simulink model "node23_case_10kV_withLoad_v2"  (R2022b)
settings: Solver=VariableStepAuto  StartTime=0.0  StopTime=10  FixedStep=1e-6  RelTol=1e-5
InitFcn:
  | sw=5;
  | Lf=1.75e-3+3.5e-3;
  | %Lf=3.5e-3;
  | %Cf=2e-4;
  | f=10;
  | Cf=15e-6;
  | % L=1.75e-3/2;
  | % X=100*pi*L;
  | % R=2*X;
  | R=0.25;X=R/0.66;
  | L=X/100/pi;
  | Z=sqrt(R^2+X^2);
  | f = 30;
  | kp1=10;
  | ki1=100;
  | kp4=20;
  | ki4=100;
  | kp16=20;
  | ki16=100;
  | % 负载参数
  | R1L=0;
  | X1L=0;
  | R2L=652.4467;
  | X2L=276.0351;
  | R3L=804.5741;
  | X3L=256.7790;
  | R4L=760.9867;
  | X4L=234.6376;
  | R5L=818.7384;
  | X5L=266.9799;
  | R6L=671.1329;
  | X6L=170.1801;
  | R7L=883.7621;
  | X7L=178.8663;
  | R8L=388.3725;
  | X8L=158.3040;
  | R9L=817.4819;
  | X9L=268.6933;
  | R10L=849.4733;
  | X10L=254.8420;
  | R11L=407.8415;
  | X11L=165.8504;
  | R12L=NaN;  % Bus 12 无 R、X 数据，用 NaN 标记
  | X12L=NaN;
  | R13L=751.2339;
  | X13L=329.8428;
  | R14L=294.0393;
  | X14L=141.6929;
  | R15L=761.9027;
  | X15L=284.3908;
  | R16L=740.4040;
  | X16L=318.2438;
  | R17L=674.5784;
  | X17L=316.4689;
  | R18L=776.7449;
  | X18L=316.6080;
  | R19L=766.0423;
  | X19L=335.7994;
  | R20L=746.0545;
  | X20L=344.3329;
  | ... (+266 lines)
libraries: spsSeriesRLCBranchLib x210, slpidlib x45, spsControlledVoltageSourceLib x30, spsThreePhaseVIMeasurementLib x24, spsPower3phInstantaneousLib x13, spsAlphaBetaZerotoabcLib x9, spsCurrentMeasurementLib x6, spsGroundLib x2, spspowerguiLib x1
(part 3 of 8)

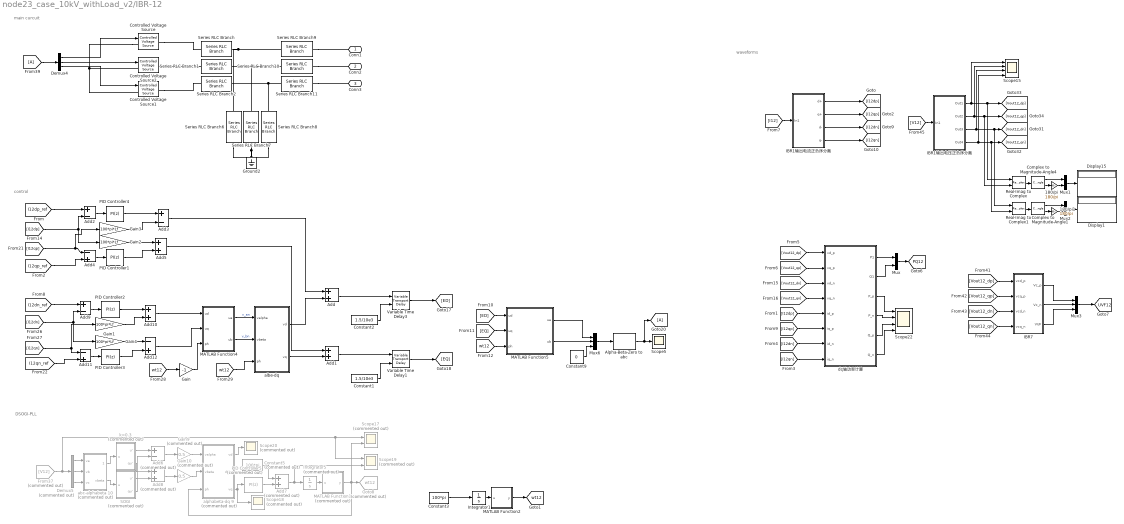
== system node23_case_10kV_withLoad_v2/IBR-12 ==
  note: waveforms
  note: DSOGI-PLL
  note: control
  note: main curcuit
  180/pi : Gain  Gain=180/pi
  180/pi1 : Gain  Gain=180/pi
  Add{,1,5,10} (4 alike) : Sum
  Add11 : Sum  Inputs=-+
  Add12 : Sum  Inputs=-+
  Add2 : Sum  Inputs=+-
  Add3 : Sum  Inputs=+-
  Add4 : Sum  Inputs=-+
  Add6 : Sum  Commented=on  Inputs=+-
  Add7 : Sum  Commented=on
  Add8 : Sum  Commented=on
  Add9 : Sum  Inputs=+-
  Alpha-Beta-Zero to abc : spsAlphaBetaZerotoabcLib/Alpha-Beta-Zero to abc
      settings: LibrarySourceBlock=|
      | sps_lib/Control/Alpha-Beta-Zero
      | to abc
  Complex to Magnitude-Angle1 : ComplexToMagnitudeAngle
  Complex to Magnitude-Angle4 : ComplexToMagnitudeAngle
  Constant1 : Constant  Value=1.5/10e3
  Constant2 : Constant  Value=1.5/10e3
  Constant3 : Constant  Value=100*pi
  Constant5 : Constant  Commented=on  Value=100*pi
  Constant9 : Constant  Value=0
  Controlled Voltage Source : spsControlledVoltageSourceLib/Controlled Voltage Source  Initialize=on  Source_Type=AC  Amplitude=0  Phase=0  Frequency=0  Measurements=None
  Controlled Voltage Source1 : spsControlledVoltageSourceLib/Controlled Voltage Source  Initialize=on  Source_Type=AC  Amplitude=0  Phase=0  Frequency=0  Measurements=None
  Controlled Voltage Source2 : spsControlledVoltageSourceLib/Controlled Voltage Source  Initialize=on  Source_Type=AC  Amplitude=0  Phase=0  Frequency=0  Measurements=None
  Demux4 : Demux  Outputs=3
  Demux5 : Demux  Commented=on  Outputs=3
  Display1 : Display
  Display15 : Display
  From37 : From  Commented=on  GotoTag=V12  TagVisibility=global
  From39 : From
  Gain : Gain  Gain=-1
  Gain{1..4} (4 alike) : Gain  Gain=100*pi*Lf
  Gain10 : Gain  Commented=on  Gain=0.5
  Gain9 : Gain  Commented=on  Gain=0.5
  Goto20 : Goto
  Goto8 : Goto  Commented=on  GotoTag=wt12  TagVisibility=global
  Ground2 : spsGroundLib/Ground  LConnTagsString=a
  IBR1输出电压正负序分离 : Subsystem
  IBR1输出电流正负序分离 : Subsystem
  IBR7 : MATLAB Function  TreatAsAtomicUnit=on
  Integrator1 : Integrator
  Integrator5 : Integrator  Commented=on
  MATLAB Function1 : MATLAB Function  Commented=on  TreatAsAtomicUnit=on
  MATLAB Function2 : MATLAB Function  TreatAsAtomicUnit=on
  MATLAB Function4 : MATLAB Function  TreatAsAtomicUnit=on
  MATLAB Function5 : MATLAB Function  TreatAsAtomicUnit=on
  Mux : Mux  Inputs=2
  Mux1 : Mux  Inputs=2
  Mux2 : Mux  Inputs=2
  Mux3 : Mux  Inputs=3
  Mux6 : Mux  Inputs=3
  PID Controller{1..4} (4 alike) : slpidlib/PID Controller  Controller=PI  Form=Parallel  TimeDomain=Discrete-time  UseExternalTs=off  SampleTime=-1  IntegratorMethod=Forward Euler  FilterMethod=Forward Euler  ControllerParametersSource=internal  P=kp1  I=ki1  UseKiTs=off  D=0  N=100  UseFilter=on  TunerSelectOption=Transfer Function Based (PID Tuner App)  InitialConditionSource=internal  InitialConditionForIntegrator=0  InitialConditionForFilter=0  DifferentiatorICPrevScaledInput=0  ExternalReset=none  TrackingMode=off  Kt=1  LimitOutput=off  SatLimitsSource=internal  UpperSaturationLimit=5  LowerSaturationLimit=-5  LinearizeAsGain=on  AntiWindupMode=none  Kb=1  LimitIntegrator=off  UpperIntegratorSaturationLimit=inf  LowerIntegratorSaturationLimit=-inf  POutMin=[]  POutMax=[]  IOutMin=[]  IOutMax=[]  DOutMin=[]  DOutMax=[]  NOutMin=[]  NOutMax=[]  SumOutMin=[]  SumOutMax=[]  SaturationOutMin=[]  SaturationOutMax=[]  PParamMin=[]  PParamMax=[]  IParamMin=[]  IParamMax=[]  DParamMin=[]  DParamMax=[]  NParamMin=[]  NParamMax=[]  KbParamMin=[]  KbParamMax=[]  KtParamMin=[]  KtParamMax=[]  KbOutMin=[]  KbOutMax=[]  KtOutMin=[]  KtOutMax=[]  IntegratorOutMin=[]  IntegratorOutMax=[]  FilterOutMin=[]  FilterOutMax=[]  SumI1OutMin=[]  SumI1OutMax=[]  SumI2OutMin=[]  SumI2OutMax=[]  SumI3OutMin=[]  SumI3OutMax=[]  SumI4OutMin=[]  SumI4OutMax=[]  SumDOutMin=[]  SumDOutMax=[]  DifferentiatorOutMin=[]  DifferentiatorOutMax=[]  FilterDiffOutCoefMin=[]  FilterDiffOutCoefMax=[]  ReciprocalOutMin=[]  ReciprocalOutMax=[]  SumDenOutMin=[]  SumDenOutMax=[]  SumNumOutMin=[]  SumNumOutMax=[]  DivideOutMin=[]  DivideOutMax=[]  UdiffTsProdOutMin=[]  UdiffTsProdOutMax=[]  NTsProdOutMin=[]  NTsProdOutMax=[]  UintegralTsProdOutMin=[]  UintegralTsProdOutMax=[]  UngainTsProdOutMin=[]  UngainTsProdOutMax=[]  ClampingZeroOutDataTypeStr=Inherit: Inherit via back propagation  ClampingZeroOutMin=[]  ClampingZeroOutMax=[]  FilterDenConstantOutDataTypeStr=Inherit: Inherit via back propagation  FilterDenConstantOutMin=[]  FilterDenConstantOutMax=[]  PCopyOutDataTypeStr=Inherit: Inherit via back propagation  PCopyOutMin=[]  PCopyOutMax=[]  NCopyOutDataTypeStr=Inherit: Inherit via back propagation  NCopyOutMin=[]  NCopyOutMax=[]  IntegratorContinuousStateAttributes=''  IntegratorStateMustResolveToSignalObject=off  IntegratorRTWStateStorageClass=Auto  FilterContinuousStateAttributes=''  FilterStateMustResolveToSignalObject=off  FilterRTWStateStorageClass=Auto  ParallelPVariant=InternalParameters  IdealPVariant=Disabled  IVariant=InternalParameters  DVariant=Disabled  IntegratorVariant=Discrete  SatVariant=Disabled  AWVariant=Passthrough  PCopyVariant=Disabled  TRVariant=Disabled  FdbkBlocksVariant=Forward  IdealPFdbkVariant=Disabled  SatFdbkVariant=Disabled  DerivativeFilterVariant=Disabled  NVariant=Disabled  NCopyVariant=Disabled_SignalSpec  FilterICVariant=Disabled  IntegratorICVariant=InternalICs  ExternalResetVariant=Disabled  TRSumVariant=Passthrough  SumFdbkVariant=Disabled  SumVariant=Sum_PI  TsampFilterVariant=InternalTs  TsampNgainVariant=Passthrough  TsampIntegralVariant=Passthrough  ExternalSaturationOutDataTypeStr=Inherit: Same as second input
  PID Controller5 : slpidlib/PID Controller  Commented=on  Controller=PI  Form=Parallel  TimeDomain=Discrete-time  UseExternalTs=off  SampleTime=-1  IntegratorMethod=Forward Euler  FilterMethod=Forward Euler  ControllerParametersSource=internal  P=1  I=3  UseKiTs=off  D=0  N=100  UseFilter=on  TunerSelectOption=Transfer Function Based (PID Tuner App)  InitialConditionSource=internal  InitialConditionForIntegrator=0  InitialConditionForFilter=0  DifferentiatorICPrevScaledInput=0  ExternalReset=none  TrackingMode=off  Kt=1  LimitOutput=off  SatLimitsSource=internal  UpperSaturationLimit=inf  LowerSaturationLimit=-inf  LinearizeAsGain=on  AntiWindupMode=none  Kb=1  LimitIntegrator=off  UpperIntegratorSaturationLimit=inf  LowerIntegratorSaturationLimit=-inf  POutMin=[]  POutMax=[]  IOutMin=[]  IOutMax=[]  DOutMin=[]  DOutMax=[]  NOutMin=[]  NOutMax=[]  SumOutMin=[]  SumOutMax=[]  SaturationOutMin=[]  SaturationOutMax=[]  PParamMin=[]  PParamMax=[]  IParamMin=[]  IParamMax=[]  DParamMin=[]  DParamMax=[]  NParamMin=[]  NParamMax=[]  KbParamMin=[]  KbParamMax=[]  KtParamMin=[]  KtParamMax=[]  KbOutMin=[]  KbOutMax=[]  KtOutMin=[]  KtOutMax=[]  IntegratorOutMin=[]  IntegratorOutMax=[]  FilterOutMin=[]  FilterOutMax=[]  SumI1OutMin=[]  SumI1OutMax=[]  SumI2OutMin=[]  SumI2OutMax=[]  SumI3OutMin=[]  SumI3OutMax=[]  SumI4OutMin=[]  SumI4OutMax=[]  SumDOutMin=[]  SumDOutMax=[]  DifferentiatorOutMin=[]  DifferentiatorOutMax=[]  FilterDiffOutCoefMin=[]  FilterDiffOutCoefMax=[]  ReciprocalOutMin=[]  ReciprocalOutMax=[]  SumDenOutMin=[]  SumDenOutMax=[]  SumNumOutMin=[]  SumNumOutMax=[]  DivideOutMin=[]  DivideOutMax=[]  UdiffTsProdOutMin=[]  UdiffTsProdOutMax=[]  NTsProdOutMin=[]  NTsProdOutMax=[]  UintegralTsProdOutMin=[]  UintegralTsProdOutMax=[]  UngainTsProdOutMin=[]  UngainTsProdOutMax=[]  ClampingZeroOutDataTypeStr=Inherit: Inherit via back propagation  ClampingZeroOutMin=[]  ClampingZeroOutMax=[]  FilterDenConstantOutDataTypeStr=Inherit: Inherit via back propagation  FilterDenConstantOutMin=[]  FilterDenConstantOutMax=[]  PCopyOutDataTypeStr=Inherit: Inherit via back propagation  PCopyOutMin=[]  PCopyOutMax=[]  NCopyOutDataTypeStr=Inherit: Inherit via back propagation  NCopyOutMin=[]  NCopyOutMax=[]  IntegratorContinuousStateAttributes=''  IntegratorStateMustResolveToSignalObject=off  IntegratorRTWStateStorageClass=Auto  FilterContinuousStateAttributes=''  FilterStateMustResolveToSignalObject=off  FilterRTWStateStorageClass=Auto  ParallelPVariant=InternalParameters  IdealPVariant=Disabled  IVariant=InternalParameters  DVariant=Disabled  IntegratorVariant=Discrete  SatVariant=Disabled  AWVariant=Passthrough  PCopyVariant=Disabled  TRVariant=Disabled  FdbkBlocksVariant=Forward  IdealPFdbkVariant=Disabled  SatFdbkVariant=Disabled  DerivativeFilterVariant=Disabled  NVariant=Disabled  NCopyVariant=Disabled_SignalSpec  FilterICVariant=Disabled  IntegratorICVariant=InternalICs  ExternalResetVariant=Disabled  TRSumVariant=Passthrough  SumFdbkVariant=Disabled  SumVariant=Sum_PI  TsampFilterVariant=InternalTs  TsampNgainVariant=Passthrough  TsampIntegralVariant=Passthrough  ExternalSaturationOutDataTypeStr=Inherit: Same as second input
  Real-Imag to Complex : RealImagToComplex
  Real-Imag to Complex1 : RealImagToComplex
  SOGI : Subsystem  Commented=on
  Scope15 : Scope  NumInputPorts=4
  Scope17 : Scope  Commented=on  NumInputPorts=2
  Scope18 : Scope  Commented=on
  Scope19 : Scope  Commented=on  NumInputPorts=2
  Scope20 : Scope  Commented=on
  Scope22 : Scope  NumInputPorts=4
  Scope5 : Scope
  Series RLC Branch : spsSeriesRLCBranchLib/Series RLC Branch  LConnTagsString=__new0  RConnTagsString=__new0  BranchType=L  Resistance=1  Inductance=3.5e-3  SetiL0=off  InitialCurrent=0  Capacitance=1e-6  Setx0=off  InitialVoltage=0  Measurements=None
  Series RLC Branch1 : spsSeriesRLCBranchLib/Series RLC Branch  LConnTagsString=__new0  RConnTagsString=__new0  BranchType=L  Resistance=1  Inductance=3.5e-3  SetiL0=off  InitialCurrent=0  Capacitance=1e-6  Setx0=off  InitialVoltage=0  Measurements=None
  Series RLC Branch10 : spsSeriesRLCBranchLib/Series RLC Branch  LConnTagsString=__new0  RConnTagsString=__new0  BranchType=L  Resistance=1  Inductance=1.75e-3  SetiL0=off  InitialCurrent=0  Capacitance=1e-6  Setx0=off  InitialVoltage=0  Measurements=None
  Series RLC Branch11 : spsSeriesRLCBranchLib/Series RLC Branch  LConnTagsString=__new0  RConnTagsString=__new0  BranchType=L  Resistance=1  Inductance=1.75e-3  SetiL0=off  InitialCurrent=0  Capacitance=1e-6  Setx0=off  InitialVoltage=0  Measurements=None
  Series RLC Branch2 : spsSeriesRLCBranchLib/Series RLC Branch  LConnTagsString=__new0  RConnTagsString=__new0  BranchType=L  Resistance=1  Inductance=3.5e-3  SetiL0=off  InitialCurrent=0  Capacitance=1e-6  Setx0=off  InitialVoltage=0  Measurements=None
  Series RLC Branch6 : spsSeriesRLCBranchLib/Series RLC Branch  LConnTagsString=__new0  RConnTagsString=__new0  BranchType=RC  Resistance=5  Inductance=500e-6  SetiL0=off  InitialCurrent=0  Capacitance=Cf  Setx0=off  InitialVoltage=0  Measurements=None
  Series RLC Branch7 : spsSeriesRLCBranchLib/Series RLC Branch  LConnTagsString=__new0  RConnTagsString=__new0  BranchType=RC  Resistance=5  Inductance=500e-6  SetiL0=off  InitialCurrent=0  Capacitance=Cf  Setx0=off  InitialVoltage=0  Measurements=None
  Series RLC Branch8 : spsSeriesRLCBranchLib/Series RLC Branch  LConnTagsString=__new0  RConnTagsString=__new0  BranchType=RC  Resistance=5  Inductance=500e-6  SetiL0=off  InitialCurrent=0  Capacitance=Cf  Setx0=off  InitialVoltage=0  Measurements=None
  Series RLC Branch9 : spsSeriesRLCBranchLib/Series RLC Branch  LConnTagsString=__new0  RConnTagsString=__new0  BranchType=L  Resistance=1  Inductance=1.75e-3  SetiL0=off  InitialCurrent=0  Capacitance=1e-6  Setx0=off  InitialVoltage=0  Measurements=None
  Variable Time Delay1 : VariableTransportDelay  MaximumDelay=10  PadeOrder=2
  Variable Time Delay3 : VariableTransportDelay  MaximumDelay=10  PadeOrder=2
  abc-alphabeta 10 : MATLAB Function  Commented=on  TreatAsAtomicUnit=on
  albe-dq : MATLAB Function  TreatAsAtomicUnit=on
  alphabeta-dq 9 : MATLAB Function  Commented=on  TreatAsAtomicUnit=on
  dq轴功率计算 : MATLAB Function  TreatAsAtomicUnit=on
  k=0.3 : Subsystem  Commented=on
  Conn1 : PMIOPort  Side=Right
  Conn2 : PMIOPort  Port=2  Side=Right
  Conn3 : PMIOPort  Port=3  Side=Right
  tag scope: PQ12=global, UVF12=global, wt12=global
  wires:
  IBR1输出电压正负序分离/4(Out4) -> [Vout12_qn], Real-Imag to Complex1/2, Scope15/4
  Complex to Magnitude-Angle1/1 -> Mux2/1
  Complex to Magnitude-Angle1/2 -> 180/pi1/1
  Real-Imag to Complex1/1 -> Complex to Magnitude-Angle1/1
  180/pi1/1 -> Mux2/2
  Mux2/1 -> Display1/1
  IBR1输出电压正负序分离/1(Out1) -> Scope15/1, [Vout12_dp], Real-Imag to Complex/1
  Mux1/1 -> Display15/1
  180/pi/1 -> Mux1/2
  Real-Imag to Complex/1 -> Complex to Magnitude-Angle4/1
  Complex to Magnitude-Angle4/2 -> 180/pi/1
  Complex to Magnitude-Angle4/1 -> Mux1/1
  Mux/1 -> [PQ12]
  [I12dn] -> dq轴功率计算/7(id_n)
  [I12qp] -> dq轴功率计算/6(iq_p)
  [I12dp] -> dq轴功率计算/5(id_p)
  [Vout12_qn] -> dq轴功率计算/4(vq_n)
  [Vout12_dn] -> dq轴功率计算/3(vd_n)
  [Vout12_qp] -> dq轴功率计算/2(vq_p)
  [I12qn] -> dq轴功率计算/8(iq_n)
  [Vout12_dp] -> dq轴功率计算/1(vd_p)
  dq轴功率计算/2(Q1) -> Mux/2
  dq轴功率计算/3(P_p) -> Scope22/1
  dq轴功率计算/5(Q_p) -> Scope22/3
  dq轴功率计算/4(P_n) -> Scope22/2
  dq轴功率计算/6(Q_n) -> Scope22/4
  dq轴功率计算/1(P1) -> Mux/1
  [wt12] -> Gain/1
  MATLAB Function4/1(ua) -> albe-dq/1(valpha)  "v_an"
  [I12qn] -> Add11/1, Gain1/1
  [I12dn] -> Gain4/1, Add9/2
  PID Controller1/1 -> Add5/2
  albe-dq/2(vq) -> Add1/2
  Gain1/1 -> Add10/2
  Add5/1 -> Add1/1
  albe-dq/1(vd) -> Add/2
  Gain2/1 -> Add5/1
  [I12qp] -> Add4/1, Gain3/1
  [wt12] -> albe-dq/3(ph)
  PID Controller4/1 -> Add3/1
  Gain3/1 -> Add3/2
  Add4/1 -> PID Controller1/1
  [ED] -> MATLAB Function5/1(ud)
  Add11/1 -> PID Controller3/1
  Add10/1 -> MATLAB Function4/1(ud)
  MATLAB Function4/2(ub) -> albe-dq/2(vbeta)  "v_bn"
  MATLAB Function5/2(ub) -> Mux6/2
  Add9/1 -> PID Controller2/1
  Gain/1 -> MATLAB Function4/3(ph)
  Gain4/1 -> Add12/1
  [I12dp] -> Add2/2, Gain2/1
  PID Controller2/1 -> Add10/1
  PID Controller3/1 -> Add12/2
  Add3/1 -> Add/1
  [wt12] -> MATLAB Function5/3(ph)
  Add12/1 -> MATLAB Function4/2(uq)
  [EQ] -> MATLAB Function5/2(uq)
  [Vout12_qn] -> IBR7/4(vcq_n)
  [Vout12_dp] -> IBR7/1(vcd_p)
  [Vout12_qp] -> IBR7/2(vcq_p)
  [Vout12_dn] -> IBR7/3(vcd_n)
  [I12] -> IBR1输出电流正负序分离/1(In1)
  IBR1输出电流正负序分离/1(d+) -> [I12dp]
  IBR1输出电压正负序分离/2(Out2) -> [Vout12_qp], Real-Imag to Complex/2, Scope15/2
  [V12] -> IBR1输出电压正负序分离/1(In1)
  IBR1输出电流正负序分离/4(q-) -> [I12qn]
  IBR1输出电压正负序分离/3(Out3) -> Scope15/3, [Vout12_dn], Real-Imag to Complex1/1
  IBR7/2(Vc_n) -> Mux3/2
  IBR7/1(Vc_p) -> Mux3/1
  IBR7/3(VUF) -> Mux3/3
  Mux3/1 -> [UVF12]
  Add2/1 -> PID Controller4/1
  MATLAB Function5/1(ua) -> Mux6/1
  Mux6/1 -> Alpha-Beta-Zero to abc/1
  Alpha-Beta-Zero to abc/1 -> Goto20/1, Scope5/1
  Constant9/1 -> Mux6/3
  From39/1 -> Demux4/1
  Demux4/2 -> Controlled Voltage Source2/1
  Demux4/3 -> Controlled Voltage Source1/1
  Demux4/1 -> Controlled Voltage Source/1
  [I12qn_ref] -> Add11/2
  [I12dn_ref] -> Add9/1
  [I12qp_ref] -> Add4/2
  [I12dp_ref] -> Add2/1
  IBR1输出电流正负序分离/2(q+) -> [I12qp]
  IBR1输出电流正负序分离/3(d-) -> [I12dn]
  Add/1 -> Variable Time Delay3/1
  Constant2/1 -> Variable Time Delay3/2
  Variable Time Delay3/1 -> [ED]
  Constant1/1 -> Variable Time Delay1/2
  Add1/1 -> Variable Time Delay1/1
  Variable Time Delay1/1 -> [EQ]
  Add8/1 -> Gain10/1
  Gain9/1 -> alphabeta-dq 9/1(valpha)
  Integrator5/1 -> MATLAB Function1/1(u)
  MATLAB Function1/1(y) -> Goto8/1, Scope17/2, alphabeta-dq 9/3(ph)
  Constant5/1 -> Add7/1
  alphabeta-dq 9/1(vd) -> Scope20/1
  From37/1 -> Scope19/1, Scope17/1, Demux5/1
  Gain10/1 -> alphabeta-dq 9/2(vbeta)
  alphabeta-dq 9/3(vq) -> PID Controller5/1, Scope18/1
  SOGI/1(u') -> Add8/2
  Add7/1 -> Integrator5/1, Scope19/2
  k=0.3/1(u') -> Add6/1
  Add6/1 -> Gain9/1
  abc-alphabeta 10/1(valpha) -> k=0.3/1(u)
  Demux5/2 -> abc-alphabeta 10/2(vb)
  Demux5/1 -> abc-alphabeta 10/1(va)
  k=0.3/2(qu') -> Add8/1
  Demux5/3 -> abc-alphabeta 10/3(vc)
  SOGI/2(qu') -> Add6/2
  abc-alphabeta 10/2(vbeta) -> SOGI/1(u)
  PID Controller5/1 -> Add7/2
  Constant3/1 -> Integrator1/1
  MATLAB Function2/1(y) -> [wt12]
  Integrator1/1 -> MATLAB Function2/1(u)
  connections:
  Series RLC Branch9/RConn1 -- Conn1/RConn1
  Series RLC Branch10/RConn1 -- Conn2/RConn1
  Series RLC Branch11/RConn1 -- Conn3/RConn1
  Controlled Voltage Source/RConn1 -- Series RLC Branch/LConn1
  Series RLC Branch8/RConn1 -- Series RLC Branch6/RConn1 -- Series RLC Branch7/RConn1 -- Ground2/LConn1
  Controlled Voltage Source1/RConn1 -- Series RLC Branch2/LConn1
  Controlled Voltage Source2/RConn1 -- Series RLC Branch1/LConn1
  Series RLC Branch9/LConn1 -- Series RLC Branch6/LConn1 -- Series RLC Branch/RConn1
  Series RLC Branch10/LConn1 -- Series RLC Branch1/RConn1 -- Series RLC Branch7/LConn1
  Series RLC Branch11/LConn1 -- Series RLC Branch2/RConn1 -- Series RLC Branch8/LConn1
  Controlled Voltage Source/LConn1 -- Controlled Voltage Source2/LConn1 -- Controlled Voltage Source1/LConn1

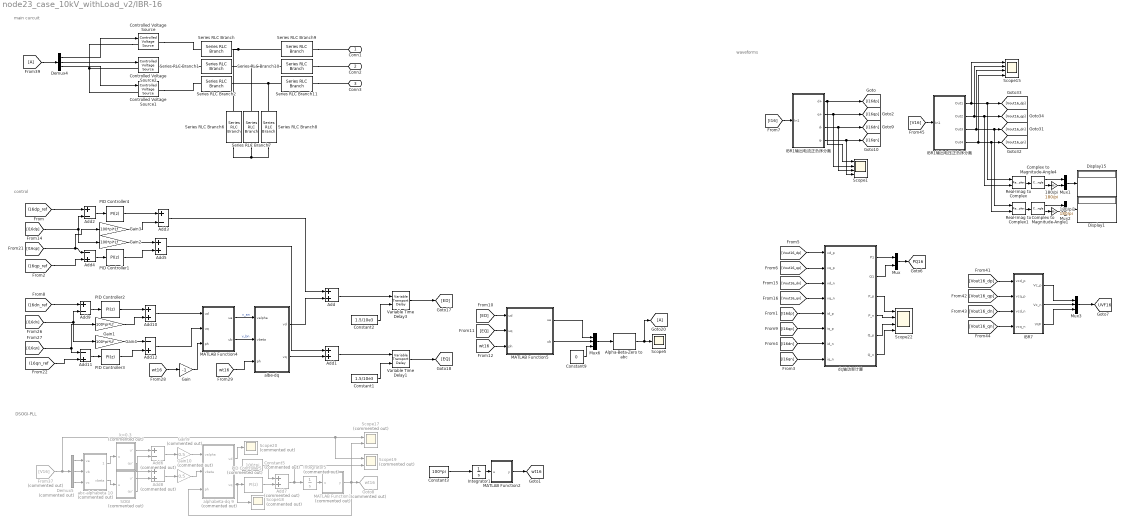
== system node23_case_10kV_withLoad_v2/IBR-16 ==
  note: waveforms
  note: DSOGI-PLL
  note: control
  note: main curcuit
  180/pi : Gain  Gain=180/pi
  180/pi1 : Gain  Gain=180/pi
  Add{,1,5,10} (4 alike) : Sum
  Add11 : Sum  Inputs=-+
  Add12 : Sum  Inputs=-+
  Add2 : Sum  Inputs=+-
  Add3 : Sum  Inputs=+-
  Add4 : Sum  Inputs=-+
  Add6 : Sum  Commented=on  Inputs=+-
  Add7 : Sum  Commented=on
  Add8 : Sum  Commented=on
  Add9 : Sum  Inputs=+-
  Alpha-Beta-Zero to abc : spsAlphaBetaZerotoabcLib/Alpha-Beta-Zero to abc
      settings: LibrarySourceBlock=|
      | sps_lib/Control/Alpha-Beta-Zero
      | to abc
  Complex to Magnitude-Angle1 : ComplexToMagnitudeAngle
  Complex to Magnitude-Angle4 : ComplexToMagnitudeAngle
  Constant1 : Constant  Value=1.5/10e3
  Constant2 : Constant  Value=1.5/10e3
  Constant3 : Constant  Value=100*pi
  Constant5 : Constant  Commented=on  Value=100*pi
  Constant9 : Constant  Value=0
  Controlled Voltage Source : spsControlledVoltageSourceLib/Controlled Voltage Source  Initialize=on  Source_Type=AC  Amplitude=0  Phase=0  Frequency=0  Measurements=None
  Controlled Voltage Source1 : spsControlledVoltageSourceLib/Controlled Voltage Source  Initialize=on  Source_Type=AC  Amplitude=0  Phase=0  Frequency=0  Measurements=None
  Controlled Voltage Source2 : spsControlledVoltageSourceLib/Controlled Voltage Source  Initialize=on  Source_Type=AC  Amplitude=0  Phase=0  Frequency=0  Measurements=None
  Demux4 : Demux  Outputs=3
  Demux5 : Demux  Commented=on  Outputs=3
  Display1 : Display
  Display15 : Display
  From37 : From  Commented=on  GotoTag=V16  TagVisibility=global
  From39 : From
  Gain : Gain  Gain=-1
  Gain{1..4} (4 alike) : Gain  Gain=100*pi*Lf
  Gain10 : Gain  Commented=on  Gain=0.5
  Gain9 : Gain  Commented=on  Gain=0.5
  Goto20 : Goto
  Goto8 : Goto  Commented=on  GotoTag=wt16  TagVisibility=global
  IBR1输出电压正负序分离 : Subsystem
  IBR1输出电流正负序分离 : Subsystem
  IBR7 : MATLAB Function  TreatAsAtomicUnit=on
  Integrator1 : Integrator
  Integrator5 : Integrator  Commented=on
  MATLAB Function1 : MATLAB Function  Commented=on  TreatAsAtomicUnit=on
  MATLAB Function2 : MATLAB Function  TreatAsAtomicUnit=on
  MATLAB Function4 : MATLAB Function  TreatAsAtomicUnit=on
  MATLAB Function5 : MATLAB Function  TreatAsAtomicUnit=on
  Mux : Mux  Inputs=2
  Mux1 : Mux  Inputs=2
  Mux2 : Mux  Inputs=2
  Mux3 : Mux  Inputs=3
  Mux6 : Mux  Inputs=3
  PID Controller{1..4} (4 alike) : slpidlib/PID Controller  Controller=PI  Form=Parallel  TimeDomain=Discrete-time  UseExternalTs=off  SampleTime=-1  IntegratorMethod=Forward Euler  FilterMethod=Forward Euler  ControllerParametersSource=internal  P=kp16  I=ki16  UseKiTs=off  D=0  N=100  UseFilter=on  TunerSelectOption=Transfer Function Based (PID Tuner App)  InitialConditionSource=internal  InitialConditionForIntegrator=0  InitialConditionForFilter=0  DifferentiatorICPrevScaledInput=0  ExternalReset=none  TrackingMode=off  Kt=1  LimitOutput=off  SatLimitsSource=internal  UpperSaturationLimit=5  LowerSaturationLimit=-5  LinearizeAsGain=on  AntiWindupMode=none  Kb=1  LimitIntegrator=off  UpperIntegratorSaturationLimit=inf  LowerIntegratorSaturationLimit=-inf  POutMin=[]  POutMax=[]  IOutMin=[]  IOutMax=[]  DOutMin=[]  DOutMax=[]  NOutMin=[]  NOutMax=[]  SumOutMin=[]  SumOutMax=[]  SaturationOutMin=[]  SaturationOutMax=[]  PParamMin=[]  PParamMax=[]  IParamMin=[]  IParamMax=[]  DParamMin=[]  DParamMax=[]  NParamMin=[]  NParamMax=[]  KbParamMin=[]  KbParamMax=[]  KtParamMin=[]  KtParamMax=[]  KbOutMin=[]  KbOutMax=[]  KtOutMin=[]  KtOutMax=[]  IntegratorOutMin=[]  IntegratorOutMax=[]  FilterOutMin=[]  FilterOutMax=[]  SumI1OutMin=[]  SumI1OutMax=[]  SumI2OutMin=[]  SumI2OutMax=[]  SumI3OutMin=[]  SumI3OutMax=[]  SumI4OutMin=[]  SumI4OutMax=[]  SumDOutMin=[]  SumDOutMax=[]  DifferentiatorOutMin=[]  DifferentiatorOutMax=[]  FilterDiffOutCoefMin=[]  FilterDiffOutCoefMax=[]  ReciprocalOutMin=[]  ReciprocalOutMax=[]  SumDenOutMin=[]  SumDenOutMax=[]  SumNumOutMin=[]  SumNumOutMax=[]  DivideOutMin=[]  DivideOutMax=[]  UdiffTsProdOutMin=[]  UdiffTsProdOutMax=[]  NTsProdOutMin=[]  NTsProdOutMax=[]  UintegralTsProdOutMin=[]  UintegralTsProdOutMax=[]  UngainTsProdOutMin=[]  UngainTsProdOutMax=[]  ClampingZeroOutDataTypeStr=Inherit: Inherit via back propagation  ClampingZeroOutMin=[]  ClampingZeroOutMax=[]  FilterDenConstantOutDataTypeStr=Inherit: Inherit via back propagation  FilterDenConstantOutMin=[]  FilterDenConstantOutMax=[]  PCopyOutDataTypeStr=Inherit: Inherit via back propagation  PCopyOutMin=[]  PCopyOutMax=[]  NCopyOutDataTypeStr=Inherit: Inherit via back propagation  NCopyOutMin=[]  NCopyOutMax=[]  IntegratorContinuousStateAttributes=''  IntegratorStateMustResolveToSignalObject=off  IntegratorRTWStateStorageClass=Auto  FilterContinuousStateAttributes=''  FilterStateMustResolveToSignalObject=off  FilterRTWStateStorageClass=Auto  ParallelPVariant=InternalParameters  IdealPVariant=Disabled  IVariant=InternalParameters  DVariant=Disabled  IntegratorVariant=Discrete  SatVariant=Disabled  AWVariant=Passthrough  PCopyVariant=Disabled  TRVariant=Disabled  FdbkBlocksVariant=Forward  IdealPFdbkVariant=Disabled  SatFdbkVariant=Disabled  DerivativeFilterVariant=Disabled  NVariant=Disabled  NCopyVariant=Disabled_SignalSpec  FilterICVariant=Disabled  IntegratorICVariant=InternalICs  ExternalResetVariant=Disabled  TRSumVariant=Passthrough  SumFdbkVariant=Disabled  SumVariant=Sum_PI  TsampFilterVariant=InternalTs  TsampNgainVariant=Passthrough  TsampIntegralVariant=Passthrough  ExternalSaturationOutDataTypeStr=Inherit: Same as second input
  PID Controller5 : slpidlib/PID Controller  Commented=on  Controller=PI  Form=Parallel  TimeDomain=Discrete-time  UseExternalTs=off  SampleTime=-1  IntegratorMethod=Forward Euler  FilterMethod=Forward Euler  ControllerParametersSource=internal  P=1  I=3  UseKiTs=off  D=0  N=100  UseFilter=on  TunerSelectOption=Transfer Function Based (PID Tuner App)  InitialConditionSource=internal  InitialConditionForIntegrator=0  InitialConditionForFilter=0  DifferentiatorICPrevScaledInput=0  ExternalReset=none  TrackingMode=off  Kt=1  LimitOutput=off  SatLimitsSource=internal  UpperSaturationLimit=inf  LowerSaturationLimit=-inf  LinearizeAsGain=on  AntiWindupMode=none  Kb=1  LimitIntegrator=off  UpperIntegratorSaturationLimit=inf  LowerIntegratorSaturationLimit=-inf  POutMin=[]  POutMax=[]  IOutMin=[]  IOutMax=[]  DOutMin=[]  DOutMax=[]  NOutMin=[]  NOutMax=[]  SumOutMin=[]  SumOutMax=[]  SaturationOutMin=[]  SaturationOutMax=[]  PParamMin=[]  PParamMax=[]  IParamMin=[]  IParamMax=[]  DParamMin=[]  DParamMax=[]  NParamMin=[]  NParamMax=[]  KbParamMin=[]  KbParamMax=[]  KtParamMin=[]  KtParamMax=[]  KbOutMin=[]  KbOutMax=[]  KtOutMin=[]  KtOutMax=[]  IntegratorOutMin=[]  IntegratorOutMax=[]  FilterOutMin=[]  FilterOutMax=[]  SumI1OutMin=[]  SumI1OutMax=[]  SumI2OutMin=[]  SumI2OutMax=[]  SumI3OutMin=[]  SumI3OutMax=[]  SumI4OutMin=[]  SumI4OutMax=[]  SumDOutMin=[]  SumDOutMax=[]  DifferentiatorOutMin=[]  DifferentiatorOutMax=[]  FilterDiffOutCoefMin=[]  FilterDiffOutCoefMax=[]  ReciprocalOutMin=[]  ReciprocalOutMax=[]  SumDenOutMin=[]  SumDenOutMax=[]  SumNumOutMin=[]  SumNumOutMax=[]  DivideOutMin=[]  DivideOutMax=[]  UdiffTsProdOutMin=[]  UdiffTsProdOutMax=[]  NTsProdOutMin=[]  NTsProdOutMax=[]  UintegralTsProdOutMin=[]  UintegralTsProdOutMax=[]  UngainTsProdOutMin=[]  UngainTsProdOutMax=[]  ClampingZeroOutDataTypeStr=Inherit: Inherit via back propagation  ClampingZeroOutMin=[]  ClampingZeroOutMax=[]  FilterDenConstantOutDataTypeStr=Inherit: Inherit via back propagation  FilterDenConstantOutMin=[]  FilterDenConstantOutMax=[]  PCopyOutDataTypeStr=Inherit: Inherit via back propagation  PCopyOutMin=[]  PCopyOutMax=[]  NCopyOutDataTypeStr=Inherit: Inherit via back propagation  NCopyOutMin=[]  NCopyOutMax=[]  IntegratorContinuousStateAttributes=''  IntegratorStateMustResolveToSignalObject=off  IntegratorRTWStateStorageClass=Auto  FilterContinuousStateAttributes=''  FilterStateMustResolveToSignalObject=off  FilterRTWStateStorageClass=Auto  ParallelPVariant=InternalParameters  IdealPVariant=Disabled  IVariant=InternalParameters  DVariant=Disabled  IntegratorVariant=Discrete  SatVariant=Disabled  AWVariant=Passthrough  PCopyVariant=Disabled  TRVariant=Disabled  FdbkBlocksVariant=Forward  IdealPFdbkVariant=Disabled  SatFdbkVariant=Disabled  DerivativeFilterVariant=Disabled  NVariant=Disabled  NCopyVariant=Disabled_SignalSpec  FilterICVariant=Disabled  IntegratorICVariant=InternalICs  ExternalResetVariant=Disabled  TRSumVariant=Passthrough  SumFdbkVariant=Disabled  SumVariant=Sum_PI  TsampFilterVariant=InternalTs  TsampNgainVariant=Passthrough  TsampIntegralVariant=Passthrough  ExternalSaturationOutDataTypeStr=Inherit: Same as second input
  Real-Imag to Complex : RealImagToComplex
  Real-Imag to Complex1 : RealImagToComplex
  SOGI : Subsystem  Commented=on
  Scope1 : Scope  NumInputPorts=4
  Scope15 : Scope  NumInputPorts=4
  Scope17 : Scope  Commented=on  NumInputPorts=2
  Scope18 : Scope  Commented=on
  Scope19 : Scope  Commented=on  NumInputPorts=2
  Scope20 : Scope  Commented=on
  Scope22 : Scope  NumInputPorts=4
  Scope5 : Scope
  Series RLC Branch : spsSeriesRLCBranchLib/Series RLC Branch  LConnTagsString=__new0  RConnTagsString=__new0  BranchType=L  Resistance=1  Inductance=3.5e-3  SetiL0=off  InitialCurrent=0  Capacitance=1e-6  Setx0=off  InitialVoltage=0  Measurements=None
  Series RLC Branch1 : spsSeriesRLCBranchLib/Series RLC Branch  LConnTagsString=__new0  RConnTagsString=__new0  BranchType=L  Resistance=1  Inductance=3.5e-3  SetiL0=off  InitialCurrent=0  Capacitance=1e-6  Setx0=off  InitialVoltage=0  Measurements=None
  Series RLC Branch10 : spsSeriesRLCBranchLib/Series RLC Branch  LConnTagsString=__new0  RConnTagsString=__new0  BranchType=L  Resistance=1  Inductance=1.75e-3  SetiL0=off  InitialCurrent=0  Capacitance=1e-6  Setx0=off  InitialVoltage=0  Measurements=None
  Series RLC Branch11 : spsSeriesRLCBranchLib/Series RLC Branch  LConnTagsString=__new0  RConnTagsString=__new0  BranchType=L  Resistance=1  Inductance=1.75e-3  SetiL0=off  InitialCurrent=0  Capacitance=1e-6  Setx0=off  InitialVoltage=0  Measurements=None
  Series RLC Branch2 : spsSeriesRLCBranchLib/Series RLC Branch  LConnTagsString=__new0  RConnTagsString=__new0  BranchType=L  Resistance=1  Inductance=3.5e-3  SetiL0=off  InitialCurrent=0  Capacitance=1e-6  Setx0=off  InitialVoltage=0  Measurements=None
  Series RLC Branch6 : spsSeriesRLCBranchLib/Series RLC Branch  LConnTagsString=__new0  RConnTagsString=__new0  BranchType=RC  Resistance=5  Inductance=500e-6  SetiL0=off  InitialCurrent=0  Capacitance=Cf  Setx0=off  InitialVoltage=0  Measurements=None
  Series RLC Branch7 : spsSeriesRLCBranchLib/Series RLC Branch  LConnTagsString=__new0  RConnTagsString=__new0  BranchType=RC  Resistance=5  Inductance=500e-6  SetiL0=off  InitialCurrent=0  Capacitance=Cf  Setx0=off  InitialVoltage=0  Measurements=None
  Series RLC Branch8 : spsSeriesRLCBranchLib/Series RLC Branch  LConnTagsString=__new0  RConnTagsString=__new0  BranchType=RC  Resistance=5  Inductance=500e-6  SetiL0=off  InitialCurrent=0  Capacitance=Cf  Setx0=off  InitialVoltage=0  Measurements=None
  Series RLC Branch9 : spsSeriesRLCBranchLib/Series RLC Branch  LConnTagsString=__new0  RConnTagsString=__new0  BranchType=L  Resistance=1  Inductance=1.75e-3  SetiL0=off  InitialCurrent=0  Capacitance=1e-6  Setx0=off  InitialVoltage=0  Measurements=None
  Variable Time Delay1 : VariableTransportDelay  MaximumDelay=10  PadeOrder=2
  Variable Time Delay3 : VariableTransportDelay  MaximumDelay=10  PadeOrder=2
  abc-alphabeta 10 : MATLAB Function  Commented=on  TreatAsAtomicUnit=on
  albe-dq : MATLAB Function  TreatAsAtomicUnit=on
  alphabeta-dq 9 : MATLAB Function  Commented=on  TreatAsAtomicUnit=on
  dq轴功率计算 : MATLAB Function  TreatAsAtomicUnit=on
  k=0.3 : Subsystem  Commented=on
  Conn1 : PMIOPort  Side=Right
  Conn2 : PMIOPort  Port=2  Side=Right
  Conn3 : PMIOPort  Port=3  Side=Right
  tag scope: PQ16=global, UVF16=global, wt16=global
  wires:
  IBR1输出电压正负序分离/4(Out4) -> [Vout16_qn], Real-Imag to Complex1/2, Scope15/4
  Complex to Magnitude-Angle1/1 -> Mux2/1
  Complex to Magnitude-Angle1/2 -> 180/pi1/1
  Real-Imag to Complex1/1 -> Complex to Magnitude-Angle1/1
  180/pi1/1 -> Mux2/2
  Mux2/1 -> Display1/1
  IBR1输出电压正负序分离/1(Out1) -> Scope15/1, [Vout16_dp], Real-Imag to Complex/1
  Mux1/1 -> Display15/1
  180/pi/1 -> Mux1/2
  Real-Imag to Complex/1 -> Complex to Magnitude-Angle4/1
  Complex to Magnitude-Angle4/2 -> 180/pi/1
  Complex to Magnitude-Angle4/1 -> Mux1/1
  Mux/1 -> [PQ16]
  [I16dn] -> dq轴功率计算/7(id_n)
  [I16qp] -> dq轴功率计算/6(iq_p)
  [I16dp] -> dq轴功率计算/5(id_p)
  [Vout16_qn] -> dq轴功率计算/4(vq_n)
  [Vout16_dn] -> dq轴功率计算/3(vd_n)
  [Vout16_qp] -> dq轴功率计算/2(vq_p)
  [I16qn] -> dq轴功率计算/8(iq_n)
  [Vout16_dp] -> dq轴功率计算/1(vd_p)
  dq轴功率计算/2(Q1) -> Mux/2
  dq轴功率计算/3(P_p) -> Scope22/1
  dq轴功率计算/5(Q_p) -> Scope22/3
  dq轴功率计算/4(P_n) -> Scope22/2
  dq轴功率计算/6(Q_n) -> Scope22/4
  dq轴功率计算/1(P1) -> Mux/1
  [wt16] -> Gain/1
  MATLAB Function4/1(ua) -> albe-dq/1(valpha)  "v_an"
  [I16qn] -> Add11/1, Gain1/1
  [I16dn] -> Gain4/1, Add9/2
  PID Controller1/1 -> Add5/2
  albe-dq/2(vq) -> Add1/2
  Gain1/1 -> Add10/2
  Add5/1 -> Add1/1
  albe-dq/1(vd) -> Add/2
  Gain2/1 -> Add5/1
  [I16qp] -> Add4/1, Gain3/1
  [wt16] -> albe-dq/3(ph)
  PID Controller4/1 -> Add3/1
  Gain3/1 -> Add3/2
  Add4/1 -> PID Controller1/1
  [ED] -> MATLAB Function5/1(ud)
  Add11/1 -> PID Controller3/1
  Add10/1 -> MATLAB Function4/1(ud)
  MATLAB Function4/2(ub) -> albe-dq/2(vbeta)  "v_bn"
  MATLAB Function5/2(ub) -> Mux6/2
  Add9/1 -> PID Controller2/1
  Gain/1 -> MATLAB Function4/3(ph)
  Gain4/1 -> Add12/1
  [I16dp] -> Add2/2, Gain2/1
  PID Controller2/1 -> Add10/1
  PID Controller3/1 -> Add12/2
  Add3/1 -> Add/1
  [wt16] -> MATLAB Function5/3(ph)
  Add12/1 -> MATLAB Function4/2(uq)
  [EQ] -> MATLAB Function5/2(uq)
  [Vout16_qn] -> IBR7/4(vcq_n)
  [Vout16_dp] -> IBR7/1(vcd_p)
  [Vout16_qp] -> IBR7/2(vcq_p)
  [Vout16_dn] -> IBR7/3(vcd_n)
  [I16] -> IBR1输出电流正负序分离/1(In1)
  IBR1输出电流正负序分离/1(d+) -> Scope1/1, [I16dp]
  IBR1输出电压正负序分离/2(Out2) -> [Vout16_qp], Real-Imag to Complex/2, Scope15/2
  [V16] -> IBR1输出电压正负序分离/1(In1)
  IBR1输出电压正负序分离/3(Out3) -> Scope15/3, [Vout16_dn], Real-Imag to Complex1/1
  IBR7/2(Vc_n) -> Mux3/2
  IBR7/1(Vc_p) -> Mux3/1
  IBR7/3(VUF) -> Mux3/3
  Mux3/1 -> [UVF16]
  Add2/1 -> PID Controller4/1
  MATLAB Function5/1(ua) -> Mux6/1
  Mux6/1 -> Alpha-Beta-Zero to abc/1
  Alpha-Beta-Zero to abc/1 -> Goto20/1, Scope5/1
  Constant9/1 -> Mux6/3
  From39/1 -> Demux4/1
  Demux4/2 -> Controlled Voltage Source2/1
  Demux4/3 -> Controlled Voltage Source1/1
  Demux4/1 -> Controlled Voltage Source/1
  [I16qn_ref] -> Add11/2
  [I16dn_ref] -> Add9/1
  [I16qp_ref] -> Add4/2
  [I16dp_ref] -> Add2/1
  IBR1输出电流正负序分离/2(q+) -> Scope1/2, [I16qp]
  Add/1 -> Variable Time Delay3/1
  Constant2/1 -> Variable Time Delay3/2
  Variable Time Delay3/1 -> [ED]
  Constant1/1 -> Variable Time Delay1/2
  Add1/1 -> Variable Time Delay1/1
  Variable Time Delay1/1 -> [EQ]
  Add8/1 -> Gain10/1
  Gain9/1 -> alphabeta-dq 9/1(valpha)
  Integrator5/1 -> MATLAB Function1/1(u)
  MATLAB Function1/1(y) -> Goto8/1, Scope17/2, alphabeta-dq 9/3(ph)
  Constant5/1 -> Add7/1
  alphabeta-dq 9/1(vd) -> Scope20/1
  From37/1 -> Scope19/1, Scope17/1, Demux5/1
  Gain10/1 -> alphabeta-dq 9/2(vbeta)
  alphabeta-dq 9/2(vq) -> Scope18/1, PID Controller5/1
  SOGI/1(u') -> Add8/2
  Add7/1 -> Integrator5/1, Scope19/2
  k=0.3/1(u') -> Add6/1
  Add6/1 -> Gain9/1
  abc-alphabeta 10/1(valpha) -> k=0.3/1(u)
  Demux5/2 -> abc-alphabeta 10/2(vb)
  Demux5/1 -> abc-alphabeta 10/1(va)
  k=0.3/2(qu') -> Add8/1
  Demux5/3 -> abc-alphabeta 10/3(vc)
  SOGI/2(qu') -> Add6/2
  abc-alphabeta 10/2(vbeta) -> SOGI/1(u)
  PID Controller5/1 -> Add7/2
  Constant3/1 -> Integrator1/1
  MATLAB Function2/1(y) -> [wt16]
  Integrator1/1 -> MATLAB Function2/1(u)
  IBR1输出电流正负序分离/3(d-) -> Scope1/3, [I16dn]
  IBR1输出电流正负序分离/4(q-) -> Scope1/4, [I16qn]
  connections:
  Series RLC Branch9/RConn1 -- Conn1/RConn1
  Series RLC Branch10/RConn1 -- Conn2/RConn1
  Series RLC Branch11/RConn1 -- Conn3/RConn1
  Controlled Voltage Source/RConn1 -- Series RLC Branch/LConn1
  Series RLC Branch8/RConn1 -- Series RLC Branch7/RConn1 -- Series RLC Branch6/RConn1
  Controlled Voltage Source1/RConn1 -- Series RLC Branch2/LConn1
  Controlled Voltage Source2/RConn1 -- Series RLC Branch1/LConn1
  Series RLC Branch9/LConn1 -- Series RLC Branch6/LConn1 -- Series RLC Branch/RConn1
  Series RLC Branch10/LConn1 -- Series RLC Branch1/RConn1 -- Series RLC Branch7/LConn1
  Series RLC Branch11/LConn1 -- Series RLC Branch2/RConn1 -- Series RLC Branch8/LConn1
  Controlled Voltage Source/LConn1 -- Controlled Voltage Source2/LConn1 -- Controlled Voltage Source1/LConn1
